simulink model "closed_loop"  (R2023b)
settings: Solver=VariableStepAuto  StartTime=0.0  StopTime=15  RelTol=1e-3
values from neighbouring files (symbols this model uses):
  Ts = 0.02    [system_configuration.m]
  u_nom = 0    [system_configuration.m]
  y_nom = [0 0]    [system_configuration.m]
libraries: cstblocks x2
settings Model: Creator=aniello  LastModifiedBy=aniello

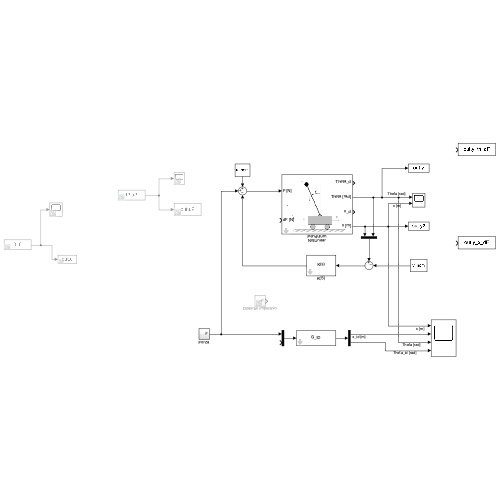
[thumbnail: Simulink's stored preview of the top-level diagram]
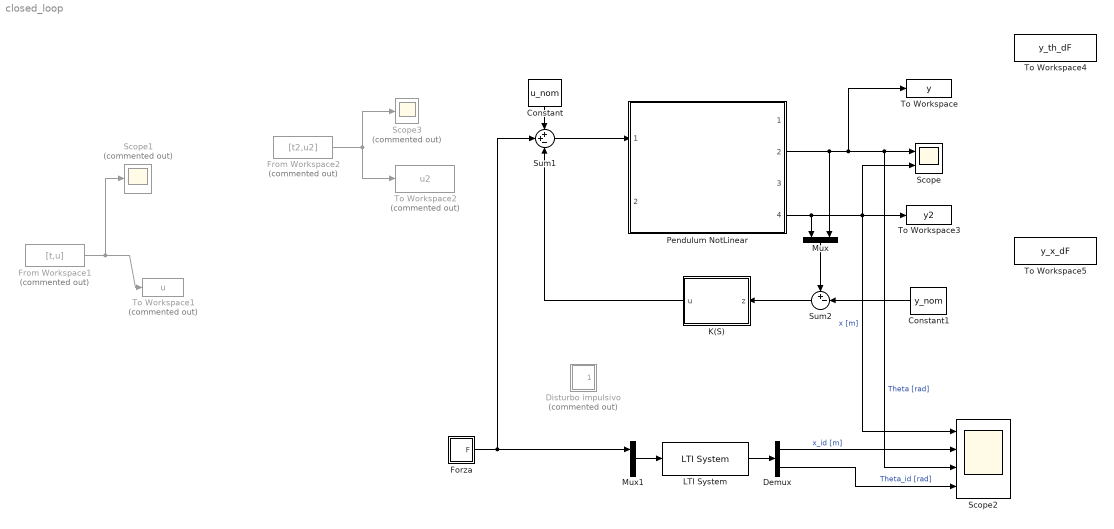
== system closed_loop ==
  Constant : Constant  Value=u_nom
  Constant1 : Constant  Value=y_nom
  Demux : Demux  Outputs=2
  Disturbo impulsivo : Subsystem  Commented=on
  Forza : Subsystem
  From Workspace1 : FromWorkspace  Commented=on  VariableName=[t,u]  Interpolate=off  OutputAfterFinalValue=Setting to zero
  From Workspace2 : FromWorkspace  Commented=on  VariableName=[t2,u2]  Interpolate=off  OutputAfterFinalValue=Setting to zero
  K(S) : Subsystem
      mask Display: disp('K(s)');
  LTI System : cstblocks/LTI System  sys=G_ID  IC=[]  PadeOrder=0
  Mux : Mux  Inputs=2
  Mux1 : Mux  Inputs=2
  Pendulum NotLinear : Subsystem  ReferencedSubsystem=pendulum
  Scope : Scope  NumInputPorts=2
  Scope1 : Scope  Commented=on
  Scope2 : Scope  NumInputPorts=4
  Scope3 : Scope  Commented=on
  Sum1 : Sum  Inputs=++-
  Sum2 : Sum  Inputs=+-|
  To Workspace : ToWorkspace  VariableName=y  SaveFormat=Structure With Time  SampleTime=Ts
  To Workspace1 : ToWorkspace  Commented=on  VariableName=u  SaveFormat=Structure With Time  SampleTime=Ts
  To Workspace2 : ToWorkspace  Commented=on  VariableName=u2  SaveFormat=Structure With Time  SampleTime=Ts
  To Workspace3 : ToWorkspace  VariableName=y2  SaveFormat=Structure With Time  SampleTime=Ts
  To Workspace4 : ToWorkspace  VariableName=y_th_dF  SaveFormat=Structure With Time  SampleTime=Ts
  To Workspace5 : ToWorkspace  VariableName=y_x_dF  SaveFormat=Structure With Time  SampleTime=Ts
  wires:
  Pendulum NotLinear/4 -> Scope2/1, Scope/2, To Workspace3/1, Mux/1  "x [m]"
  Sum1/1 -> Pendulum NotLinear/1
  K(S)/1(u) -> Sum1/3
  Constant1/1 -> Sum2/2
  Constant/1 -> Sum1/1
  Pendulum NotLinear/2 -> Scope2/3, Scope/1, To Workspace/1, Mux/2  "Theta [rad]"
  From Workspace1/1 -> To Workspace1/1, Scope1/1
  From Workspace2/1 -> Scope3/1, To Workspace2/1
  Mux/1 -> Sum2/1
  Sum2/1 -> K(S)/1(z)
  Mux1/1 -> LTI System/1
  LTI System/1 -> Demux/1
  Demux/2 -> Scope2/4  "Theta_id [rad]"
  Demux/1 -> Scope2/2  "x_id [m]"
  Forza/1(F) -> Sum1/2, Mux1/1

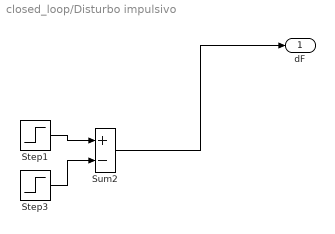
== system closed_loop/Disturbo impulsivo ==
  Step1 : Step  Time=2  SampleTime=0
  Step3 : Step  Time=2.01  SampleTime=0
  Sum2 : Sum  Inputs=+-
  dF : Outport
  wires:
  Sum2/1 -> dF/1
  Step3/1 -> Sum2/2
  Step1/1 -> Sum2/1

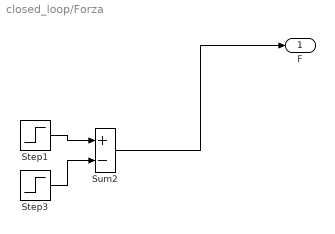
== system closed_loop/Forza ==
  Step1 : Step  SampleTime=0
  Step3 : Step  Time=1.1  SampleTime=0
  Sum2 : Sum  Inputs=+-
  F : Outport
  wires:
  Step1/1 -> Sum2/1
  Step3/1 -> Sum2/2
  Sum2/1 -> F/1

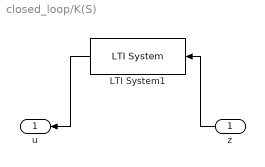
== system closed_loop/K(S) ==
  z : Inport
  LTI System1 : cstblocks/LTI System  sys=K_s  IC=[]  PadeOrder=0
  u : Outport
  wires:
  LTI System1/1 -> u/1
  z/1 -> LTI System1/1
